simulink model "KMeanClustering"  (R2016a)
settings: Solver=VariableStepAuto  StartTime=0.0  StopTime=10.0  RelTol=1e-3
undefined symbols (not defined in the file): Rec, SDTV
libraries: visionsinks x10, visionconversions x5, visionsources x3, visionanalysis x3
settings Model: Creator=YASARA  LastModifiedBy=YASARA

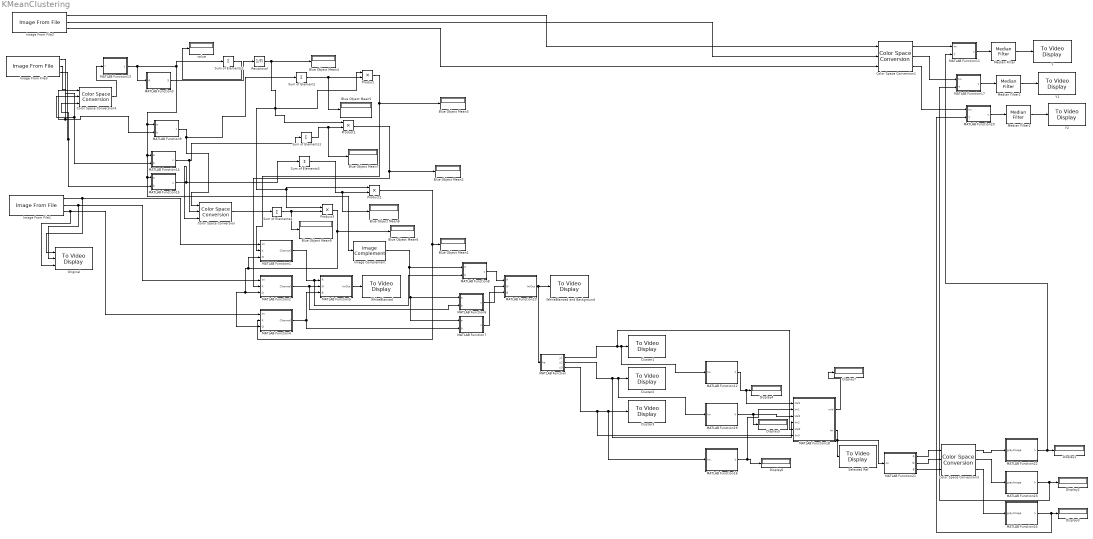
== system KMeanClustering ==
  Blue Object Mean{1..9} (9 alike) : Display
  Cluster1 : visionsinks/To Video Display  windowSizeMode=Normal  openAtMdlStart=on  fullScreen=off  videoWindowX=875  videoWindowY=150  saveWindowSize=off  videoWindowWidth=512  videoWindowHeight=384  inputColorFormat=RGB  inputType=Obsolete  imagePorts=One multidimensional signal  OutputDevice=On-screen video monitor  dataOrg=Column-major  isWindowOpen=off
  Cluster2 : visionsinks/To Video Display  windowSizeMode=Normal  openAtMdlStart=on  fullScreen=off  videoWindowX=388  videoWindowY=306  saveWindowSize=off  videoWindowWidth=512  videoWindowHeight=384  inputColorFormat=RGB  inputType=Obsolete  imagePorts=One multidimensional signal  OutputDevice=On-screen video monitor  dataOrg=Column-major  isWindowOpen=off
  Cluster3 : visionsinks/To Video Display  windowSizeMode=Normal  openAtMdlStart=on  fullScreen=off  videoWindowX=-29  videoWindowY=257  saveWindowSize=off  videoWindowWidth=512  videoWindowHeight=384  inputColorFormat=RGB  inputType=Obsolete  imagePorts=One multidimensional signal  OutputDevice=On-screen video monitor  dataOrg=Column-major  isWindowOpen=off
  Color Space Conversion : visionconversions/Color Space  Conversion  conversion=Obsolete  conversionActive=R'G'B' to intensity  wp_str=D65  rec=Rec. 601 (SDTV)  sys=1125/60/2:1  imagePorts=Separate color signals
  Color Space Conversion1 : visionconversions/Color Space  Conversion  conversion=Obsolete  conversionActive=R'G'B' to Y'CbCr  wp_str=D65  rec=Rec. 601 (SDTV)  sys=1125/60/2:1  imagePorts=Separate color signals
  Color Space Conversion3 : visionconversions/Color Space  Conversion  conversion=Obsolete  conversionActive=R'G'B' to Y'CbCr  wp_str=D65  rec=Rec. 601 (SDTV)  sys=1125/60/2:1  imagePorts=Separate color signals
  Color Space Conversion4 : visionconversions/Color Space  Conversion  conversion=Obsolete  conversionActive=R'G'B' to intensity  wp_str=D65  rec=Rec. 601 (SDTV)  sys=1125/60/2:1  imagePorts=Separate color signals
  Display{1..7} (7 alike) : Display
  Image Complement : visionconversions/Image Complement
  Image From File1 : visionsources/Image From File  Tag=vipblks_nd  FileName=C:\Users\YASARA\Desktop\FYPReview\New folder\Stem_Leaf\DSC_1206.JPG  imagePorts=Separate color signals  Ts=1  ImageDataType=uint8  Signed=on  WordLength=16  sdImageDataType=uint(8)  FractionLengthMode=User-defined  FractionLength=15  OutPortLabels=R|G|B
  Image From File2 : visionsources/Image From File  Tag=vipblks_nd  FileName=C:\Users\YASARA\Desktop\FYPReview\New folder\Stem_Leaf\DSC_1206.JPG  imagePorts=Separate color signals  Ts=1  ImageDataType=uint8  Signed=on  WordLength=16  sdImageDataType=uint(8)  FractionLengthMode=User-defined  FractionLength=15  OutPortLabels=R|G|B
  Image From File3 : visionsources/Image From File  Tag=vipblks_nd  FileName=C:\Users\YASARA\Desktop\FYPReview\New folder\Stem_Leaf\DSC_1206.JPG  imagePorts=Separate color signals  Ts=1  ImageDataType=double  Signed=on  WordLength=16  sdImageDataType=uint(8)  FractionLengthMode=User-defined  FractionLength=15  OutPortLabels=R|G|B
  MATLAB Function : MATLAB Function  TreatAsAtomicUnit=on
  MATLAB Function1 : MATLAB Function  TreatAsAtomicUnit=on
  MATLAB Function10 : MATLAB Function  TreatAsAtomicUnit=on
  MATLAB Function11 : MATLAB Function  TreatAsAtomicUnit=on
  MATLAB Function12 : MATLAB Function  TreatAsAtomicUnit=on
  MATLAB Function13 : MATLAB Function  TreatAsAtomicUnit=on
  MATLAB Function14 : MATLAB Function  TreatAsAtomicUnit=on
  MATLAB Function15 : MATLAB Function  TreatAsAtomicUnit=on
  MATLAB Function16 : MATLAB Function  TreatAsAtomicUnit=on
  MATLAB Function17 : MATLAB Function  TreatAsAtomicUnit=on
  MATLAB Function18 : MATLAB Function  TreatAsAtomicUnit=on
  MATLAB Function19 : MATLAB Function  TreatAsAtomicUnit=on
  MATLAB Function2 : MATLAB Function  TreatAsAtomicUnit=on
  MATLAB Function20 : MATLAB Function  TreatAsAtomicUnit=on
  MATLAB Function21 : MATLAB Function  TreatAsAtomicUnit=on
  MATLAB Function22 : MATLAB Function  TreatAsAtomicUnit=on
  MATLAB Function23 : MATLAB Function  TreatAsAtomicUnit=on
  MATLAB Function24 : MATLAB Function  TreatAsAtomicUnit=on
  MATLAB Function3 : MATLAB Function  TreatAsAtomicUnit=on
  MATLAB Function4 : MATLAB Function  TreatAsAtomicUnit=on
  MATLAB Function5 : MATLAB Function  TreatAsAtomicUnit=on
  MATLAB Function6 : MATLAB Function  TreatAsAtomicUnit=on
  MATLAB Function7 : MATLAB Function  TreatAsAtomicUnit=on
  MATLAB Function8 : MATLAB Function  TreatAsAtomicUnit=on
  MATLAB Function9 : MATLAB Function  TreatAsAtomicUnit=on
  Median Filter : visionanalysis/Median Filter  nghbood=[11 11]  outSize=Same as input port I  padType=Symmetric  padSrc=Specify via dialog  padVal=0  roundingMode=Floor  overflowMode=off
  Median Filter1 : visionanalysis/Median Filter  nghbood=[11 11]  outSize=Same as input port I  padType=Symmetric  padSrc=Specify via dialog  padVal=0  roundingMode=Floor  overflowMode=off
  Median Filter2 : visionanalysis/Median Filter  nghbood=[11 11]  outSize=Same as input port I  padType=Symmetric  padSrc=Specify via dialog  padVal=0  roundingMode=Floor  overflowMode=off
  Original : visionsinks/To Video Display  windowSizeMode=Normal  openAtMdlStart=on  fullScreen=off  videoWindowX=252  videoWindowY=213  saveWindowSize=off  videoWindowWidth=512  videoWindowHeight=384  inputColorFormat=RGB  inputType=Obsolete  imagePorts=Separate color signals  OutputDevice=On-screen video monitor  dataOrg=Column-major  isWindowOpen=off
  Product{,1..3} (4 alike) : Product  OutDataTypeStr=uint8
  Reciprocal : Product  Inputs=/  OutDataTypeStr=double  SaturateOnIntegerOverflow=on  RndMeth=Zero
  Selected Ref : visionsinks/To Video Display  windowSizeMode=Normal  openAtMdlStart=on  fullScreen=off  videoWindowX=252  videoWindowY=213  saveWindowSize=off  videoWindowWidth=512  videoWindowHeight=384  inputColorFormat=RGB  inputType=Obsolete  imagePorts=One multidimensional signal  OutputDevice=On-screen video monitor  dataOrg=Column-major  isWindowOpen=off
  Sum of Elements{,1..4} (5 alike) : Sum  Inputs=+
  WhiteBlanced : visionsinks/To Video Display  windowSizeMode=Normal  openAtMdlStart=on  fullScreen=off  videoWindowX=252  videoWindowY=213  saveWindowSize=off  videoWindowWidth=512  videoWindowHeight=384  inputColorFormat=RGB  inputType=Obsolete  imagePorts=One multidimensional signal  OutputDevice=On-screen video monitor  dataOrg=Column-major  isWindowOpen=off
  WhiteBlanced and Background : visionsinks/To Video Display  windowSizeMode=Normal  openAtMdlStart=on  fullScreen=off  videoWindowX=252  videoWindowY=213  saveWindowSize=off  videoWindowWidth=512  videoWindowHeight=384  inputColorFormat=RGB  inputType=Obsolete  imagePorts=One multidimensional signal  OutputDevice=On-screen video monitor  dataOrg=Column-major  isWindowOpen=off
  Y : visionsinks/To Video Display  windowSizeMode=Normal  openAtMdlStart=on  fullScreen=off  videoWindowX=536805376  videoWindowY=536805376  saveWindowSize=off  videoWindowWidth=640  videoWindowHeight=480  inputColorFormat=RGB  inputType=Obsolete  imagePorts=One multidimensional signal  OutputDevice=On-screen video monitor  dataOrg=Column-major  isWindowOpen=off
  Y1 : visionsinks/To Video Display  windowSizeMode=Normal  openAtMdlStart=on  fullScreen=off  videoWindowX=536805376  videoWindowY=536805376  saveWindowSize=off  videoWindowWidth=640  videoWindowHeight=480  inputColorFormat=RGB  inputType=Obsolete  imagePorts=One multidimensional signal  OutputDevice=On-screen video monitor  dataOrg=Column-major  isWindowOpen=off
  Y2 : visionsinks/To Video Display  windowSizeMode=Normal  openAtMdlStart=on  fullScreen=off  videoWindowX=536805376  videoWindowY=536805376  saveWindowSize=off  videoWindowWidth=640  videoWindowHeight=480  inputColorFormat=RGB  inputType=Obsolete  imagePorts=One multidimensional signal  OutputDevice=On-screen video monitor  dataOrg=Column-major  isWindowOpen=off
  value : Display
  wires:
  Color Space Conversion4/1 -> MATLAB Function13/1(I)
  MATLAB Function9/1(c) -> Color Space Conversion/1, Sum of Elements/1
  MATLAB Function14/1(c) -> Sum of Elements1/1, Color Space Conversion/2
  MATLAB Function15/1(c) -> Sum of Elements3/1, Color Space Conversion/3
  Reciprocal/1 -> Product1/1, Product3/1, Product2/1, Product/1, Blue Object Mean4/1
  MATLAB Function13/1(y) -> MATLAB Function3/1(A), Image Complement/1, MATLAB Function15/1(a), MATLAB Function14/1(a), MATLAB Function9/1(a), Sum of Elements2/1
  Image From File3/1 -> MATLAB Function9/2(b), Color Space Conversion4/1
  Image From File3/2 -> MATLAB Function14/2(b), Color Space Conversion4/2
  Image From File3/3 -> Color Space Conversion4/3, MATLAB Function15/2(b)
  Image From File1/2 -> Original/2, MATLAB Function2/1(Im)
  Image From File1/3 -> Original/3, MATLAB Function4/1(Im)
  Product/1 -> MATLAB Function1/2(K), Blue Object Mean3/1
  Product1/1 -> Blue Object Mean2/1, MATLAB Function2/2(K)
  Product2/1 -> MATLAB Function4/2(K), Blue Object Mean1/1
  Color Space Conversion/1 -> Sum of Elements4/1
  Sum of Elements/1 -> Blue Object Mean5/1, Product/2
  Product3/1 -> Blue Object Mean6/1, MATLAB Function4/3(G), MATLAB Function2/3(G), MATLAB Function1/3(G)
  Sum of Elements1/1 -> Blue Object Mean7/1, Product1/2
  Sum of Elements3/1 -> Blue Object Mean8/1, Product2/2
  Sum of Elements4/1 -> Blue Object Mean9/1, Product3/2
  Sum of Elements2/1 -> value/1
  MATLAB Function3/1(S) -> Reciprocal/1
  MATLAB Function2/1(Channel) -> MATLAB Function6/2(b), MATLAB Function5/2(G)
  MATLAB Function4/1(Channel) -> MATLAB Function5/3(B), MATLAB Function7/2(b)
  MATLAB Function5/1(ImOut) -> WhiteBlanced/1
  MATLAB Function1/1(Channel) -> MATLAB Function8/2(b), MATLAB Function5/1(R)
  Image From File1/1 -> Original/1, MATLAB Function1/1(Im)
  Image Complement/1 -> MATLAB Function7/1(a), MATLAB Function6/1(a), MATLAB Function8/1(a)
  MATLAB Function10/1(ImOut) -> MATLAB Function/1(he), WhiteBlanced and Background/1
  MATLAB Function8/1(c) -> MATLAB Function10/1(R)
  MATLAB Function6/1(c) -> MATLAB Function10/2(G)
  MATLAB Function7/1(c) -> MATLAB Function10/3(B)
  MATLAB Function/1(y1) -> MATLAB Function18/2(Im1), MATLAB Function12/1(Im), Cluster1/1
  MATLAB Function12/1(k) -> MATLAB Function18/1(Val1), Display4/1
  MATLAB Function/2(y2) -> MATLAB Function18/4(Im2), MATLAB Function19/1(Im), Cluster2/1
  MATLAB Function19/1(k) -> MATLAB Function18/5(Val3), Display5/1
  MATLAB Function/3(y3) -> MATLAB Function18/6(Im3), MATLAB Function16/1(Im), Cluster3/1
  MATLAB Function16/1(k) -> MATLAB Function18/3(Val2), Display6/1
  MATLAB Function18/1(mid) -> Display7/1
  Median Filter/1 -> Y/1
  MATLAB Function11/1(c) -> Median Filter/1
  Color Space Conversion1/1 -> MATLAB Function11/1(Im)
  Median Filter1/1 -> Y1/1
  MATLAB Function17/1(c) -> Median Filter1/1
  Color Space Conversion1/2 -> MATLAB Function17/1(Im)
  Median Filter2/1 -> Y2/1
  MATLAB Function20/1(c) -> Median Filter2/1
  Color Space Conversion1/3 -> MATLAB Function20/1(Im)
  MATLAB Function18/2(Im) -> MATLAB Function21/1(Im), Selected Ref/1
  MATLAB Function21/1(R) -> Color Space Conversion3/1
  MATLAB Function21/2(G) -> Color Space Conversion3/2
  MATLAB Function21/3(B) -> Color Space Conversion3/3
  Color Space Conversion3/1 -> MATLAB Function22/1(grayImage)
  Color Space Conversion3/2 -> MATLAB Function23/1(grayImage)
  Color Space Conversion3/3 -> MATLAB Function24/1(grayImage)
  MATLAB Function22/1(k) -> MATLAB Function11/2(T), Display1/1
  MATLAB Function24/1(k) -> MATLAB Function20/2(T), Display3/1
  MATLAB Function23/1(k) -> MATLAB Function17/2(T), Display2/1
  Image From File2/3 -> Color Space Conversion1/3
  Image From File2/2 -> Color Space Conversion1/2
  Image From File2/1 -> Color Space Conversion1/1

== matlab function KMeanClustering/MATLAB Function1 ==
  data: Im input; K input; Channel output; G input
function Channel = fcn(Im,K,G)
Channel = uint8(double(Im) *double(G)/double(K));
return

== matlab function KMeanClustering/MATLAB Function2 ==
  data: Im input; K input; Channel output; G input
function Channel = fcn(Im,K,G)
Channel = uint8(double(Im) *double(G)/double(K));
return

== matlab function KMeanClustering/MATLAB Function3 ==
  data: A input; S output
function S = fcn(A)
%#codegen
S = sum(A(:))/100;

== matlab function KMeanClustering/MATLAB Function4 ==
  data: Im input; K input; Channel output; G input
function Channel = fcn(Im,K,G)
Channel = uint8(double(Im) *double(G)/double(K));
return

== matlab function KMeanClustering/MATLAB Function5 ==
  data: R input; G input; B input; ImOut output
function ImOut = fcn(R,G,B)
ImOut = cat(3, R, G, B);
return

== matlab function KMeanClustering/MATLAB Function6 ==
  data: a input; b input; c output
function c = fcn(a,b)
%#codegen
%c=logical(a).*double(b);
c=uint8(a).*uint8(b);

== matlab function KMeanClustering/MATLAB Function7 ==
  data: a input; b input; c output
function c = fcn(a,b)
%#codegen
%c=logical(a).*double(b);
c=uint8(a).*uint8(b);

== matlab function KMeanClustering/MATLAB Function8 ==
  data: a input; b input; c output
function c = fcn(a,b)
%#codegen
c=uint8(a).*uint8(b);
%c=uint8(b);

== matlab function KMeanClustering/MATLAB Function10 ==
  data: R input; G input; B input; ImOut output
function ImOut = fcn(R,G,B)
ImOut = cat(3, R, G, B);
return

== matlab function KMeanClustering/MATLAB Function14 ==
  data: a input; b input; c output
function c = fcn(a,b)
%#codegen
c=a.*b;
return

== matlab function KMeanClustering/MATLAB Function11 ==
  data: Im input; T input; c output
function c = fcn(Im,T)
coder.extrinsic('im2bw');
c=uint8(Im(:,:,1));
c=uint8(im2bw(Im,double(T/255)));

== matlab function KMeanClustering/MATLAB Function ==
  data: he input; y1 output; y2 output; y3 output
function [y1,y2,y3] = fcn(he)
coder.extrinsic('makecform');
cform = makecform('srgb2lab');
coder.extrinsic('applycform');
coder.extrinsic('image');
lab_he = (applycform(he,cform));
u=size(he);
p =(zeros(u(1),u(2),3));
p=im2double(lab_he);
R=p(:,:,1);
G=p(:,:,2);
B=p(:,:,3);
GB=(zeros(u(1),u(2),2));
GB=cat(3,G,B);
ab=(zeros(u(1),u(2),2));
ab =double(GB);
nrows = size(ab,1);
ncols = size(ab,2);
ab = reshape(ab,nrows*ncols,2);
nColors = 3;
[cluster_idx, cluster_center] = kmeans(ab,nColors,'distance','sqEuclidean', ...
                                      'Replicates',3);
pixel_labels = reshape(cluster_idx,nrows,ncols);       
segmented_images = cell(1,3);
rgb_label = repmat(pixel_labels,[1 1 3]);
for k = 1:nColors
    color = he;
    color(rgb_label~=k) = 0;
    %color(rgb_label ~= k) = 0;
    segmented_images{k} = color;
end
y1 = segmented_images{1};
y2 = segmented_images{2};
y3 = segmented_images{3};

== matlab function KMeanClustering/MATLAB Function12 ==
  data: Im input; k output
function k = fcn(Im)
grayImage=rgb2gray(Im);
coder.extrinsic('graythresh');
bw=logical(grayImage);
level = graythresh(grayImage);
bw = im2bw(grayImage,double(level));
k=50.0;
%bw=grayImage;
%thresh = multithresh(grayImage,2);
%bw = imquantize(grayImage,thresh);%im2bw(uint8(grayImage));

% negate the image so that the objects are white, and close the holes

bw2 = imclose(~bw,strel('disk',4));
nl=1;
% label each object
coder.extrinsic('bwlabeln');
imL=double(grayImage);
[imL,nl] = bwlabeln(bw2);
% loop through the objects to find the mean intensity values
objave=double(zeros(1,100000));
objave=reshape(objave,[1,100000]);

n=1;
%objvals=grayImage;

for n=1:nl
      A=find(imL==n);
      B=reshape(A,1,[]);
     objvals = grayImage(B);
      objave(n) = double(mean(objvals(:)));

end

k=double(sum(objave(:))/nl);

== matlab function KMeanClustering/MATLAB Function13 ==
  data: I input; y output
function y = fcn(I)
%#codegen
y=I;
 coder.extrinsic('graythresh');
level = graythresh(I);
BW = double(im2bw(I,level));
y = BW;

== matlab function KMeanClustering/MATLAB Function15 ==
  data: a input; b input; c output
function c = fcn(a,b)
%#codegen
c=a.*b;
return

== matlab function KMeanClustering/MATLAB Function9 ==
  data: a input; b input; c output
function c = fcn(a,b)
%#codegen
c=a.*b;
return

== matlab function KMeanClustering/MATLAB Function16 ==
  data: Im input; k output
function k = fcn(Im)
grayImage=rgb2gray(Im);
coder.extrinsic('graythresh');
bw=logical(grayImage);
level = graythresh(grayImage);
bw = im2bw(grayImage,double(level));
k=50.0;
%bw=grayImage;
%thresh = multithresh(grayImage,2);
%bw = imquantize(grayImage,thresh);%im2bw(uint8(grayImage));

% negate the image so that the objects are white, and close the holes

bw2 = imclose(~bw,strel('disk',4));
nl=1;
% label each object
coder.extrinsic('bwlabeln');
imL=double(grayImage);
[imL,nl] = bwlabeln(bw2);
% loop through the objects to find the mean intensity values
objave=double(zeros(1,100000));
objave=reshape(objave,[1,100000]);

n=1;
%objvals=grayImage;

for n=1:nl
      A=find(imL==n);
      B=reshape(A,1,[]);
     objvals = grayImage(B);
      objave(n) = double(mean(objvals(:)));

end

k=double(sum(objave(:))/nl);

== matlab function KMeanClustering/MATLAB Function17 ==
  data: Im input; T input; c output
function c = fcn(Im,T)
%#codegen
coder.extrinsic('im2bw');
c=uint8(Im(:,:,1));
c=uint8(im2bw(Im,double(T/255)));

== matlab function KMeanClustering/MATLAB Function18 ==
  data: Val1 input; Im1 input; mid output; Val2 input; Im2 input; Val3 input; Im3 input; Im output
function [mid,Im] = fcn(Val1,Im1,Val2,Im2,Val3,Im3)
A=[Val1,Val2,Val3];
B = sort(A);
mid=B(2);
if Val1==mid
    Im=Im1;
elseif Val2==mid
    Im=Im2;
else 
    Im=Im3;
end

== matlab function KMeanClustering/MATLAB Function19 ==
  data: Im input; k output
function k = fcn(Im)
grayImage=rgb2gray(Im);
coder.extrinsic('graythresh');
bw=logical(grayImage);
level = graythresh(grayImage);
bw = im2bw(grayImage,double(level));
k=50.0;
%bw=grayImage;
%thresh = multithresh(grayImage,2);
%bw = imquantize(grayImage,thresh);%im2bw(uint8(grayImage));

% negate the image so that the objects are white, and close the holes

bw2 = imclose(~bw,strel('disk',4));
nl=1;
% label each object
coder.extrinsic('bwlabeln');
imL=double(grayImage);
[imL,nl] = bwlabeln(bw2);
% loop through the objects to find the mean intensity values
objave=double(zeros(1,100000));
objave=reshape(objave,[1,100000]);

n=1;
%objvals=grayImage;

for n=1:nl
      A=find(imL==n);
      B=reshape(A,1,[]);
     objvals = grayImage(B);
      objave(n) = double(mean(objvals(:)));

end

k=double(sum(objave(:))/nl);

== matlab function KMeanClustering/MATLAB Function20 ==
  data: Im input; T input; c output
function c = fcn(Im,T)
%#codegen
coder.extrinsic('im2bw');
c=uint8(Im(:,:,1));
c=uint8(im2bw(Im,double(T/255)));
%c=uint8(b);

== matlab function KMeanClustering/MATLAB Function21 ==
  data: Im input; R output; G output; B output
function [R,G,B] = fcn(Im)
R=Im(:,:,1);
G=Im(:,:,2);
B=Im(:,:,3);

== matlab function KMeanClustering/MATLAB Function22 ==
  data: grayImage input; k output
function k = fcn(grayImage)
coder.extrinsic('graythresh');
bw=logical(grayImage);
level = graythresh(grayImage);
bw = im2bw(grayImage,double(level));
k=50.0;
%bw=grayImage;
%thresh = multithresh(grayImage,2);
%bw = imquantize(grayImage,thresh);%im2bw(uint8(grayImage));

% negate the image so that the objects are white, and close the holes

bw2 = imclose(~bw,strel('disk',4));
nl=1;
% label each object
coder.extrinsic('bwlabeln');
imL=double(grayImage);
[imL,nl] = bwlabeln(bw2);
% loop through the objects to find the mean intensity values
objave=double(zeros(1,100000));
objave=reshape(objave,[1,100000]);

n=1;
%objvals=grayImage;

for n=1:nl
      A=find(imL==n);
      B=reshape(A,1,[]);
     objvals = grayImage(B);
      objave(n) = double(mean(objvals(:)));

end

k=double(sum(objave(:))/nl);

== matlab function KMeanClustering/MATLAB Function23 ==
  data: grayImage input; k output
function k = fcn(grayImage)

coder.extrinsic('graythresh');
bw=logical(grayImage);
level = graythresh(grayImage);
bw = im2bw(grayImage,double(level));
k=50.0;
%bw=grayImage;
%thresh = multithresh(grayImage,2);
%bw = imquantize(grayImage,thresh);%im2bw(uint8(grayImage));

% negate the image so that the objects are white, and close the holes

bw2 = imclose(~bw,strel('disk',4));
nl=1;
% label each object
coder.extrinsic('bwlabeln');
imL=double(grayImage);
[imL,nl] = bwlabeln(bw2);
% loop through the objects to find the mean intensity values
objave=double(zeros(1,100000));
objave=reshape(objave,[1,100000]);

n=1;
%objvals=grayImage;

for n=1:nl
      A=find(imL==n);
      B=reshape(A,1,[]);
     objvals = grayImage(B);
      objave(n) = double(mean(objvals(:)));

end

k=double(sum(objave(:))/nl);

== matlab function KMeanClustering/MATLAB Function24 ==
  data: grayImage input; k output
function k = fcn(grayImage)

coder.extrinsic('graythresh');
bw=logical(grayImage);
level = graythresh(grayImage);
bw = im2bw(grayImage,double(level));
k=50.0;
%bw=grayImage;
%thresh = multithresh(grayImage,2);
%bw = imquantize(grayImage,thresh);%im2bw(uint8(grayImage));

% negate the image so that the objects are white, and close the holes

bw2 = imclose(~bw,strel('disk',4));
nl=1;
% label each object
coder.extrinsic('bwlabeln');
imL=double(grayImage);
[imL,nl] = bwlabeln(bw2);
% loop through the objects to find the mean intensity values
objave=double(zeros(1,100000));
objave=reshape(objave,[1,100000]);

n=1;
%objvals=grayImage;

for n=1:nl
      A=find(imL==n);
      B=reshape(A,1,[]);
     objvals = grayImage(B);
      objave(n) = double(mean(objvals(:)));

end

k=double(sum(objave(:))/nl);
